simulink model "roundNDecPlaces"  (R2018b)
settings: Solver=VariableStepAuto  StartTime=0.0  StopTime=10.0  RelTol=1e-3
settings Model: Creator=mcobb  LastModifiedBy=mcobb

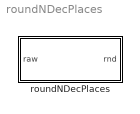
== system roundNDecPlaces ==
  roundNDecPlaces : Subsystem  mask{N=1}
      mask help: Block to round to N decimal places.

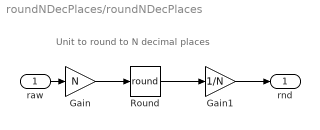
== system roundNDecPlaces/roundNDecPlaces ==
  note: Unit to round to N decimal places
  raw : Inport
  Gain : Gain  Gain=N
  Gain1 : Gain  Gain=1/N
  Round : Rounding  Operator=round
  rnd : Outport
  wires:
  raw/1 -> Gain/1
  Gain/1 -> Round/1
  Round/1 -> Gain1/1
  Gain1/1 -> rnd/1
